simulink model "BalanceCode_MSM_Micro_20b"  (R2020b)
settings: Solver=FixedStepDiscrete  StartTime=0.0  StopTime=inf  FixedStep=TS  RelTol=1e-3  EnableMultiTasking=on
PostLoadFcn:
  | TS=.007;
undefined symbols (not defined in the file): DiscIntNeverNeededParam
libraries: arduinolib x5, svdutilitieslib x4, MinSegLibrary_MinSegMega x4, RASPlib x3, simulink x3
settings Model: FPTRunName=FPA_Reference  SimulationMode=external  SILPILModeSetting=veronly  ExtModeTrigDuration=2  Creator=Alec  LastModifiedBy=hurstj
settings DataIOCC: LimitDataPoints=on  SaveFormat=Array  ReturnWorkspaceOutputs=off
settings OptimizationCC: EnhancedBackFolding=on  PassReuseOutputArgsThreshold=0  ExpressionDepthLimit=2147483647  MaxStackSize=64  OptimizeBlockOrder=speed  DifferentSizesBufferReuse=on  OptimizationCustomize=off
settings DebuggingCC: UnderspecifiedInitializationDetection=Classic  MergeDetectMultiDrivingBlocksExec=none  ParameterPrecisionLossMsg=none  ParameterTunabilityLossMsg=error  StateNameClashWarn=warning  SFUnexpectedBacktrackingDiag=warning  SFNoUnconditionalDefaultTransitionDiag=warning  SFExecutionAtInitializationDiag=none  ArithmeticOperatorsInVariantConditions=warning
settings HardwareCC: ProdBitPerInt=16  ProdBitPerPointer=16  ProdBitPerSizeT=16  ProdBitPerPtrDiffT=16  ProdLargestAtomicFloat=None  ProdWordSize=8  ProdHWDeviceType=Atmel->AVR  UseEmbeddedCoderFeatures=off  UseSimulinkCoderFeatures=off
settings ModelReferenceCC: PropagateSignalLabelsOutOfModel=off
settings SFSimCC: SimUseLocalCustomCode=off  MATLABDynamicMemAlloc=off  CustomCodeUndefinedFunction=UseInterfaceOnly
settings RTWCC: Description=Embedded Coder  SystemTargetFile=ert.tlc  HardwareBoard=Arduino Mega 2560  TemplateMakefile=ert_default_tmf  RTWVerbose=off  RTWUseLocalCustomCode=off  Toolchain=Arduino AVR  BuildConfiguration=Faster Runs
settings CodeAppCC: ForceParamTrailComments=on  OperatorAnnotations=on
settings ERTTargetCC: ERTCustomFileBanners=off  SupportContinuousTime=on  SupportNonInlinedSFcns=on  RemoveResetFunc=off  SupportVariableSizeSignals=on  ModelStepFunctionPrototypeControlCompliant=off  ExtModeStaticAllocSize=2048
settings ConfigComp: CovMetricSettings=dw  CovSaveCumulativeToWorkspaceVar=on  CovSaveSingleToWorkspaceVar=on  CovExternalEMLEnable=off

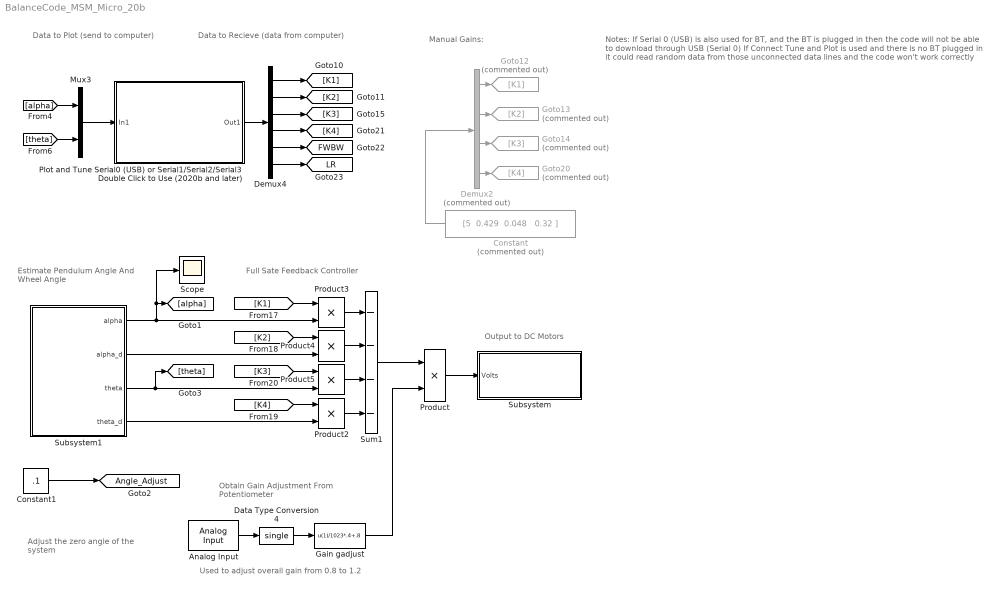
== system BalanceCode_MSM_Micro_20b ==
  note: Notes:
      |
      | If Serial 0 (USB) is also used for BT, and the BT is plugged in then the code will not be able to download through USB (Serial 0)
      |
      | If Connect Tune and Plot is used and there is no BT plugged in it could read random data from those unconnected data lines and the code won't work correctly
  note: Estimate Pendulum Angle
      | And Wheel Angle
  note: Full Sate Feedback Controller
  note: Manual Gains:
  note: Obtain Gain Adjustment
      | From Potentiometer
  note: Output to DC Motors
  note: Used to adjust overall gain from 0.8 to 1.2
  note: Adjust the zero angle
      | of the system
  note: Data to Plot
      | (send to computer)
  note: Data to Recieve
      | (data from computer)
  Analog Input : arduinolib/Analog Input  pinNumber=13  ReadResultsOnly=off  ConversionTriggerSource=Software  ExternalTriggerType=uint32( 0 )  OutputDataType=uint16  EnableConversionCompleteNotify=off  EnableOuputStatus=off  SampleTime=-1  blockPlatform=arduino
  Constant : Constant  Commented=on  Value="[5  0.429  0.048   0.32 ]"  OutDataTypeStr=single
  Constant1 : Constant  Value=.1
  Data Type Conversion4 : DataTypeConversion  OutDataTypeStr=single
  Demux2 : Demux  Commented=on
  Demux4 : Demux  Outputs=6
  Gain gadjust : Fcn  Expr=u(1)/1023*.4+.8
  Goto12 : Goto  Commented=on  GotoTag=K1
  Goto13 : Goto  Commented=on  GotoTag=K2
  Goto14 : Goto  Commented=on  GotoTag=K3
  Goto20 : Goto  Commented=on  GotoTag=K4
  Mux3 : Mux  Inputs=2
  Plot and Tune Serial0 (USB) or Serial1/Serial2/Serial3 Double Click to Use (2020b and later) : Subsystem  mask{COMport=6, Ard_Serial=3, ConnectText=<<<<<  CONNECTED  >>>>>><<<<<  CONNECTED  >>>>>><<<<<  CONNECTED  >>>>>><<<<<  CONNECTED  >>>>>>, NData=6, Data0=[7.73  0.42  0.048  0.32  0  0], DSend=[7.73  0.42  0.048  0.32  0  0], Ncx=2, NumSamples=500, Parameter10=10, Parameter12=10, Parameter13=}
      mask prompts: COMport "COM Port: (device manager)"; Ard_Serial "Arduino Serial: (0 - 3)"; NData "#  Variables:"; Data0 "Initial Values:"; DSend "Data to Send:"; Ncx "# Variables:"; NumSamples "# Samples:"; Parameter10 "OnSettingChange"; Parameter12 "OnSettingChange 2"; Parameter13 "MSM9V:  [4.8341    0.2684    0.03    0.2 0 0]*0"
      mask Callback DSend: evalin('base','if(exist(''COMdevice'')),write(COMdevice,str2num(get_param(gcb,''Dsend'')),"single"),end')
      mask Callback Parameter10: set_param(gcb,'Parameter10','10')
      mask Callback Parameter12: set_param(gcb,'Parameter12','10')
      mask DialogControl DescGroupVar Prompt: Send data to/from computer to COM device.
      mask DialogControl Control9 Prompt: Connect to COM device (Microcontroller or BT).  Can press TAB to send data in the Data to Send dialog box.  Arduino Serial 0 is USB
      mask DialogControl Control3 Prompt: Connect to COM port
      mask DialogControl Control3 Callback:
      | if(evalin('base','exist(''COMdevice'')')),
      |     disp('COM port already connected');
      | else
      |    evalin('base','COMdevice=serialport([''COM'' get_param(gcb,''COMport'')],115200)')
      | end
      | set_param(gcb,'Parameter10','1')
      mask DialogControl Control6 Prompt: Disconnect COM port
      mask DialogControl Control6 Callback:
      | evalin('base','if(exist(''COMdevice'')), disp(''Closing COM port''),clear(''COMdevice''),end')
      | set_param(gcb,'Parameter10','0')
      mask DialogControl ParameterGroupVar Prompt: Tune/Recieve - Properties of Data from Computer to Microcontroller (single data type only):
      mask DialogControl Control2 Prompt: Click to Send Data
      mask DialogControl Control2 Callback:
      | %evalin('base','write(COMdevice,30,"single")')
      | evalin('base','write(COMdevice,str2num(get_param(gcb,''Dsend'')),"single")')
      mask DialogControl Container7 Prompt: Plot/Save - Properties of Data from Microntroller to Plot/Save (single data type only)
      mask DialogControl Control7 Prompt: Click to Plot Data
      mask DialogControl Control7 Callback:
      | evalin('base','if(exist(''COMdevice'')), disp(''COM port open''),else, disp(''Opening COM Port''),end')
      | set_param(gcb,'Parameter12','10') % force mask draw
      | SerialPlot_20b_Timer(['COM' get_param(gcb,'COMport')], 'single', str2num(get_param(gcb,'NumSamples')), 115200,str2num(get_param(gcb,'Ncx')))
      | set_param(gcb,'Parameter12','11') % force mask draw
      mask DialogControl Control12 Prompt: [19 0.7 0 .19]
      mask Display:
      | text(15,75,'Serial Connect Tune')
      | text(45,60,'and Plot')
      | text(35,36,'Serial Status:')
      | 
      | if(evalin('base','exist(''COMdevice'')'))
      | 
      |     patch([0 0 300 300], [0 300 300 0],[0 1 0])
      |     text(15,75,'Serial Connect Tune')
      |     text(45,60,'and Plot')
      |     text(35,36,'Serial Status:')
      |     text(0,16,'<<<  CONNECTED  >>>>')
      |     %set_param(gcb,'ConnectText','<<<<<  CONNECTED  >>>>>><<<<<  CONNECTED  >>>>>><<<<<  CONNECTED  >>>>>><<<<<  CONNECTED  >>>>>>')
      | 
      | else
      |     text(4,16,'- - - - disconnected - - - -')
      |     %set_param(gcb,'ConnectText','- - - - - - disconnected - - - - - -- - - - - - disconnected - - - - - -- - - - - - disconnected - - - - - -- - - - - - disconnected - - - - - -- - - - - - disconnected - - - - - -')
      | end
  Product : Product  RndMeth=Zero
  Product{2..5} (4 alike) : Product
  Scope : Scope
  Subsystem : Subsystem  mask{Vsupply=7.8}
      mask prompts: Vsupply "Driver Supply Voltage"
      mask DialogControl DescGroupVar Prompt: Voltage to Motor
      mask DialogControl DescTextVar Prompt: Applies the same voltage to both motors.  No Independent control available.
      mask DialogControl ParameterGroupVar Prompt: Parameters:
      mask DialogControl Control2 Prompt: Voltage available to motor driver.  Reasonable values are 4.9 for USB, and 7.6 for a 9V battery.
      mask Display:
      | %fprintf('Volts to')
      | %fprintf(['\n\n Motors'])
      | text(35,35, 'Volts to Motor')
      | text(35,20,['Vsupply=' num2str(Vsupply)])
  Subsystem1 : Subsystem  mask{GBiasMask=0}
      mask prompts: GBiasMask "Gyro Bias (0 will calibrate automatically)"
      mask DialogControl DescGroupVar Prompt: Estimate Pendulum and Wheel Angle
      mask DialogControl DescTextVar Prompt: Estimate pendulum angle from gyroscope and acclerometer using complimentary filter.  Absolute wheel position and velocity from Encoder and Pendulum.
      mask DialogControl ParameterGroupVar Prompt: Parameters (Fixed, Non-Editable)
      mask Display:
      | fprintf('State')
      | fprintf(['\n\n Estimation'])
  Sum1 : Sum  Inputs=----
  tag scope: Angle_Adjust=global, FWBW=global, LR=global
  wires:
  Product2/1 -> Sum1/4
  Product3/1 -> Sum1/1
  Gain gadjust/1 -> Product/2
  Constant/1 -> Demux2/1
  Analog Input/1 -> Data Type Conversion4/1
  Demux2/1 -> Goto12/1
  Demux2/2 -> Goto13/1
  Product4/1 -> Sum1/2
  Data Type Conversion4/1 -> Gain gadjust/1
  Subsystem1/4(theta_d) -> Product2/2
  [K1] -> Product3/1
  Demux2/3 -> Goto14/1
  Sum1/1 -> Product/1
  Product5/1 -> Sum1/3
  [K4] -> Product2/1
  [K3] -> Product5/1
  Subsystem1/3(theta) -> [theta], Product5/2
  Demux2/4 -> Goto20/1
  [K2] -> Product4/1
  Subsystem1/2(alpha_d) -> Product4/2
  Constant1/1 -> [Angle_Adjust]
  Product/1 -> Subsystem/1(Volts)
  Subsystem1/1(alpha) -> Product3/2, Scope/1, [alpha]
  [theta] -> Mux3/2
  [alpha] -> Mux3/1
  Mux3/1 -> Plot and Tune Serial0 (USB) or Serial1/Serial2/Serial3 Double Click to Use (2020b and later)/1(In1)
  Plot and Tune Serial0 (USB) or Serial1/Serial2/Serial3 Double Click to Use (2020b and later)/1(Out1) -> Demux4/1
  Demux4/6 -> [LR]
  Demux4/1 -> [K1]
  Demux4/2 -> [K2]
  Demux4/3 -> [K3]
  Demux4/4 -> [K4]
  Demux4/5 -> [FWBW]

== system BalanceCode_MSM_Micro_20b/Plot and Tune Serial0 (USB) or Serial1//Serial2//Serial3 Double Click to Use (2020b and later) ==
  In1 : Inport
  MATLAB System : RASPlib/Double Click to Plot Serial Data/MATLAB System  is_post_2015a=~verLessThan( 'matlab', '8.6' )
      settings: SourceProductName=Rensselaer Arduino Support Package
  Send/Recieve to Serial0/Serial1/Serial2/Serial3 : Subsystem  Variant=on
  Terminator : Terminator
  Out1 : Outport
  wires:
  MATLAB System/1 -> Terminator/1
  In1/1 -> Send/Recieve to Serial0/Serial1/Serial2/Serial3/1(In1)
  Send/Recieve to Serial0/Serial1/Serial2/Serial3/1(Out1) -> Out1/1

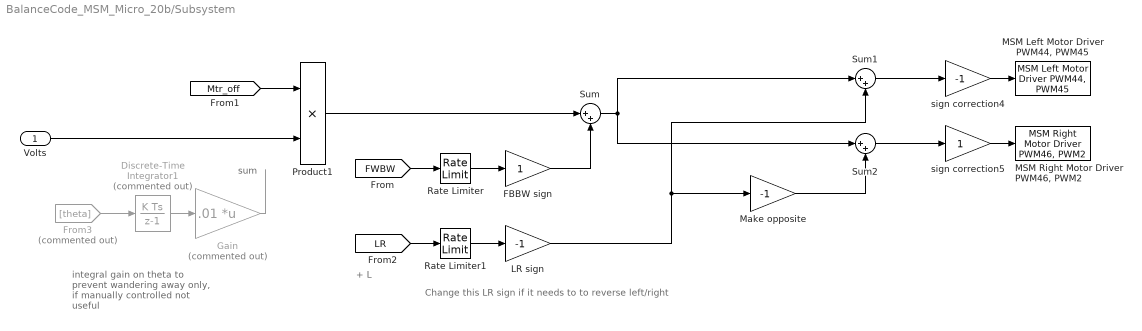
== system BalanceCode_MSM_Micro_20b/Subsystem ==
  note: sum
  note: integral gain on theta to prevent wandering away only, if manually controlled not useful
  note: Change this LR sign if it needs to to reverse left/right
  note: + L
  Volts : Inport
  Discrete-Time Integrator1 : DiscreteIntegrator  Commented=on  SampleTime=TS  ICPrevOutput=DiscIntNeverNeededParam  ICPrevScaledInput=DiscIntNeverNeededParam
  FBBW sign : Gain  OutDataTypeStr=single
  From3 : From  Commented=on  GotoTag=theta
  Gain : Gain  Commented=on  Gain=.01  Multiplication=Matrix(K*u)
  LR sign : Gain  Gain=-1  OutDataTypeStr=single
  "MSM Left Motor Driver PWM44, PWM45" : MinSegLibrary_MinSegMega/MSM Left Motor Driver PWM44, PWM45  Vsupply=Vsupply  PWMoffset=0
      settings: SourceProductName=Rensselaer Arduino Support Package
  "MSM Right Motor Driver PWM46, PWM2 " : MinSegLibrary_MinSegMega/MSM Right Motor Driver PWM46, PWM2   Vsupply=Vsupply  PWMoffset=0
      settings: SourceProductName=Rensselaer Arduino Support Package
  "Make opposite " : Gain  Gain=-1  OutDataTypeStr=single
  Product1 : Product  RndMeth=Zero
  Rate Limiter : RateLimiter  RisingSlewLimit=2  FallingSlewLimit=-2  SampleTimeMode=inherited
  Rate Limiter1 : RateLimiter  RisingSlewLimit=2  FallingSlewLimit=-2  SampleTimeMode=inherited
  Sum : Sum  Inputs=|++
  Sum1 : Sum  Inputs=|++
  Sum2 : Sum  Inputs=|++
  sign correction4 : Gain  Gain=-1  OutDataTypeStr=single
  sign correction5 : Gain  OutDataTypeStr=single
  wires:
  Volts/1 -> Product1/2
  From3/1 -> Discrete-Time Integrator1/1
  Gain/1 -> ?
  [Mtr_off] -> Product1/1
  Discrete-Time Integrator1/1 -> Gain/1
  Product1/1 -> Sum/1
  [FWBW] -> Rate Limiter/1
  Rate Limiter/1 -> FBBW sign/1
  [LR] -> Rate Limiter1/1
  Rate Limiter1/1 -> LR sign/1
  Sum/1 -> Sum2/1, Sum1/1
  sign correction5/1 -> "MSM Right Motor Driver PWM46, PWM2 "/1
  sign correction4/1 -> "MSM Left Motor Driver PWM44, PWM45"/1
  Sum1/1 -> sign correction4/1
  Sum2/1 -> sign correction5/1
  "Make opposite "/1 -> Sum2/2
  LR sign/1 -> "Make opposite "/1, Sum1/2
  FBBW sign/1 -> Sum/2

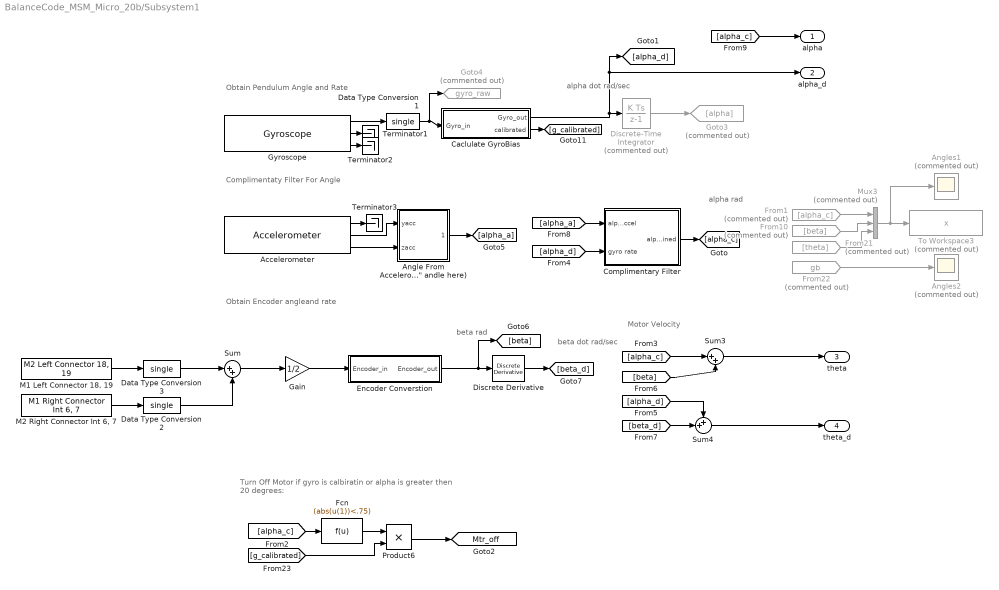
== system BalanceCode_MSM_Micro_20b/Subsystem1 ==
  note: Complimentaty Filter For Angle
  note: alpha dot
      | rad/sec
  note: alpha
      | rad
  note: Motor Velocity
  note: Turn Off Motor if gyro is calbiratin or
      | alpha is greater then 20 degrees:
  note: Obtain Pendulum Angle and Rate
  note: beta dot
      | rad/sec
  note: beta
      | rad
  note: Obtain Encoder angleand rate
  " Complimentary Filter" : Subsystem
  Accelerometer : RASPlib/Accelerometer  SimulateUsing=Code generation
      settings: SourceProductName=Rensselaer Arduino Support Package
  "Angle From Accelerometer (adjust \"zero\" andle here)" : Subsystem
  Angles1 : Scope  Commented=on
  Angles2 : Scope  Commented=on
  Caclulate GyroBias : Subsystem  mask{GSm=.00013316}
      mask DialogControl DescGroupVar Prompt: Calibrate Gyroscope
      mask DialogControl DescTextVar Prompt: Estimates gyro bias from during fist 1 second of operation.  It is important that the system is NOT moving during the fist 1 second.
      mask DialogControl ParameterGroupVar Prompt: Paramters (non tunable):
      mask DialogControl Control2 Prompt: Gyro Bias (Calibrated Automatically)
      mask DialogControl Control3 Prompt: Unit Conversion (Fixed)
  Data Type Conversion1 : DataTypeConversion  OutDataTypeStr=single
  Data Type Conversion2 : DataTypeConversion  OutDataTypeStr=single
  Data Type Conversion3 : DataTypeConversion  OutDataTypeStr=single
  Discrete Derivative : simulink/Discrete/Discrete Derivative  gainval=1.0  ICPrevScaledInput=0.0  OutMin=[]  OutMax=[]  OutDataType=fixdt(1, 16)  OutScaling=2^-10  DoSatur=off
  Discrete-Time Integrator : DiscreteIntegrator  Commented=on  SampleTime=TS  ICPrevOutput=DiscIntNeverNeededParam  ICPrevScaledInput=DiscIntNeverNeededParam
  Encoder Converstion : Subsystem  mask{ESm=0.0047}
      mask DialogControl DescGroupVar Prompt: Encoder Unit Converstion
      mask DialogControl ParameterGroupVar Prompt: Paramters (non tunable):
      mask DialogControl Control2 Prompt: Unit Conversion (Fixed)
  Fcn : Fcn  Expr=(abs(u(1))<.75)
  From1 : From  Commented=on  GotoTag=alpha_c
  From10 : From  Commented=on  GotoTag=beta
  From21 : From  Commented=on  GotoTag=theta  TagVisibility=global
  From22 : From  Commented=on  GotoTag=gb  TagVisibility=global
  Gain : Gain  Gain=1/2
  Goto3 : Goto  Commented=on  GotoTag=alpha
  Goto4 : Goto  Commented=on  GotoTag=gyro_raw  TagVisibility=global
  Gyroscope : RASPlib/Gyroscope  DLPFmode=0
      settings: SourceProductName=Rensselaer Arduino Support Package
  "M1 Left Connector 18, 19" : MinSegLibrary_MinSegMega/M2 Left Connector 18, 19  Encoder=1  PinA=18  PinB=19
      settings: SourceProductName=Rensselaer Arduino Support Package
  "M2 Right Connector Int 6, 7" : MinSegLibrary_MinSegMega/M1 Right Connector Int 6, 7  Encoder=2  PinA=6  PinB=7
      settings: SourceProductName=Rensselaer Arduino Support Package
  Mux3 : Mux  Commented=on  Inputs=3
  Product6 : Product
  Sum : Sum  Inputs=|++
  Sum3 : Sum  Inputs=|++
  Sum4 : Sum  Inputs=++|
  Terminator1 : Terminator
  Terminator2 : Terminator
  Terminator3 : Terminator
  To Workspace3 : ToWorkspace  Commented=on  VariableName=x  SampleTime=-1
      settings: Save2DSignal=2-D array (concatenate along first dimension)
  alpha : Outport
  alpha_d : Outport  Port=2
  theta : Outport  Port=3
  theta_d : Outport  Port=4
  tag scope: Mtr_off=global
  wires:
  Gyroscope/1 -> Data Type Conversion1/1
  [beta] -> Sum3/2
  Gyroscope/3 -> Terminator2/1
  [alpha_d] -> Sum4/1
  From1/1 -> Mux3/1
  Gyroscope/2 -> Terminator1/1
  [beta_d] -> Sum4/2
  [alpha_c] -> Sum3/1
  "Angle From Accelerometer (adjust \"zero\" andle here)"/1(angle rad) -> [alpha_a]
  Data Type Conversion1/1 -> Goto4/1, Caclulate GyroBias/1(Gyro_in)
  Accelerometer/3 -> "Angle From Accelerometer (adjust \"zero\" andle here)"/2(zacc)
  Discrete-Time Integrator/1 -> Goto3/1
  [alpha_a] -> " Complimentary Filter"/1(alpha accel)
  From10/1 -> Mux3/2
  From21/1 -> Mux3/3
  Accelerometer/2 -> "Angle From Accelerometer (adjust \"zero\" andle here)"/1(yacc)
  Accelerometer/1 -> Terminator3/1
  Mux3/1 -> Angles1/1, To Workspace3/1
  Caclulate GyroBias/1(Gyro_out) -> [alpha_d], alpha_d/1, Discrete-Time Integrator/1
  [alpha_d] -> " Complimentary Filter"/2(gyro rate)
  From22/1 -> Angles2/1
  Sum4/1 -> theta_d/1
  Sum3/1 -> theta/1
  Fcn/1 -> Product6/1
  Product6/1 -> [Mtr_off]
  [alpha_c] -> Fcn/1
  [g_calibrated] -> Product6/2
  Discrete Derivative/1 -> [beta_d]
  "M1 Left Connector 18, 19"/1 -> Data Type Conversion3/1
  " Complimentary Filter"/1(alpha combined) -> [alpha_c]
  [alpha_c] -> alpha/1
  Encoder Converstion/1(Encoder_out) -> [beta], Discrete Derivative/1
  Caclulate GyroBias/2(calibrated) -> [g_calibrated]
  "M2 Right Connector Int 6, 7"/1 -> Data Type Conversion2/1
  Data Type Conversion3/1 -> Sum/1
  Data Type Conversion2/1 -> Sum/2
  Sum/1 -> Gain/1
  Gain/1 -> Encoder Converstion/1(Encoder_in)

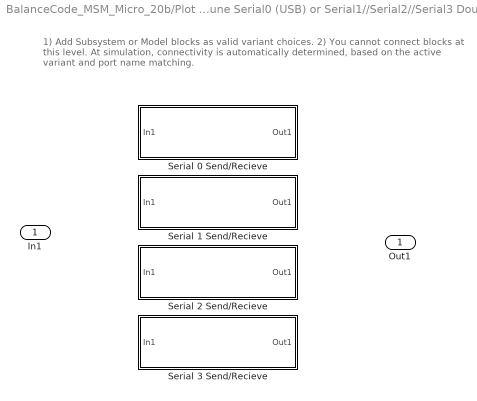
== system BalanceCode_MSM_Micro_20b/Plot and Tune Serial0 (USB) or Serial1//Serial2//Serial3 Double Click to Use (2020b and later)/Send//Recieve to Serial0//Serial1//Serial2//Serial3 ==
  note: 1) Add Subsystem or Model blocks as valid variant choices.
      | 2) You cannot connect blocks at this level. At simulation, connectivity is automatically
      | determined, based on the active variant and port name matching.
  In1 : Inport
  Serial 0 Send/Recieve : Subsystem  VariantControl=Ard_Serial==0
  Serial 1 Send/Recieve : Subsystem  VariantControl=Ard_Serial==1
  Serial 2 Send/Recieve : Subsystem  VariantControl=Ard_Serial==2
  Serial 3 Send/Recieve : Subsystem  VariantControl=Ard_Serial==3
  Out1 : Outport

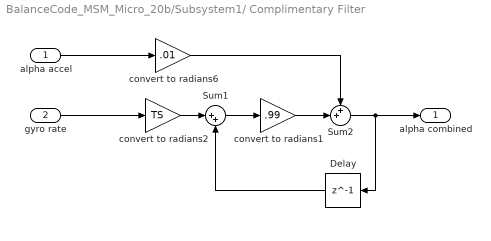
== system BalanceCode_MSM_Micro_20b/Subsystem1/ Complimentary Filter ==
  alpha accel : Inport
  gyro rate : Inport  Port=2
  Delay : Delay  DelayLength=1  SampleTime=TS
  Sum1 : Sum  Inputs=|++
  Sum2 : Sum  Inputs=++|
  convert to radians1 : Gain  Gain=.99  OutDataTypeStr=single
  convert to radians2 : Gain  Gain=TS  OutDataTypeStr=single
  convert to radians6 : Gain  Gain=.01  OutDataTypeStr=single
  alpha combined : Outport
  wires:
  gyro rate/1 -> convert to radians2/1
  Sum1/1 -> convert to radians1/1
  convert to radians6/1 -> Sum2/1
  alpha accel/1 -> convert to radians6/1
  convert to radians1/1 -> Sum2/2
  Delay/1 -> Sum1/2
  convert to radians2/1 -> Sum1/1
  Sum2/1 -> Delay/1, alpha combined/1

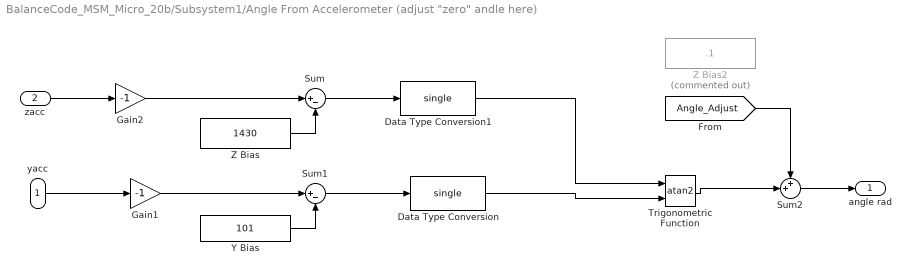
== system BalanceCode_MSM_Micro_20b/Subsystem1/Angle From Accelerometer (adjust "zero" andle here) ==
  yacc : Inport
  zacc : Inport  Port=2
  Data Type Conversion : DataTypeConversion  OutDataTypeStr=single
  Data Type Conversion1 : DataTypeConversion  OutDataTypeStr=single
  Gain1 : Gain  Gain=-1
  Gain2 : Gain  Gain=-1
  Sum : Sum  Inputs=|+-
  Sum1 : Sum  Inputs=|+-
  Sum2 : Sum  Inputs=++|
  Trigonometric Function : Trigonometry  Operator=atan2
  Y Bias : Constant  Value=101
  Z Bias : Constant  Value=1430
  Z Bias2 : Constant  Commented=on  Value=.1  OutDataTypeStr=single
  angle rad : Outport
  wires:
  Sum1/1 -> Data Type Conversion/1
  Gain2/1 -> Sum/1
  Sum/1 -> Data Type Conversion1/1
  Z Bias/1 -> Sum/2
  Gain1/1 -> Sum1/1
  Y Bias/1 -> Sum1/2
  zacc/1 -> Gain2/1
  yacc/1 -> Gain1/1
  Trigonometric Function/1 -> Sum2/2
  Sum2/1 -> angle rad/1
  [Angle_Adjust] -> Sum2/1
  Data Type Conversion1/1 -> Trigonometric Function/1
  Data Type Conversion/1 -> Trigonometric Function/2

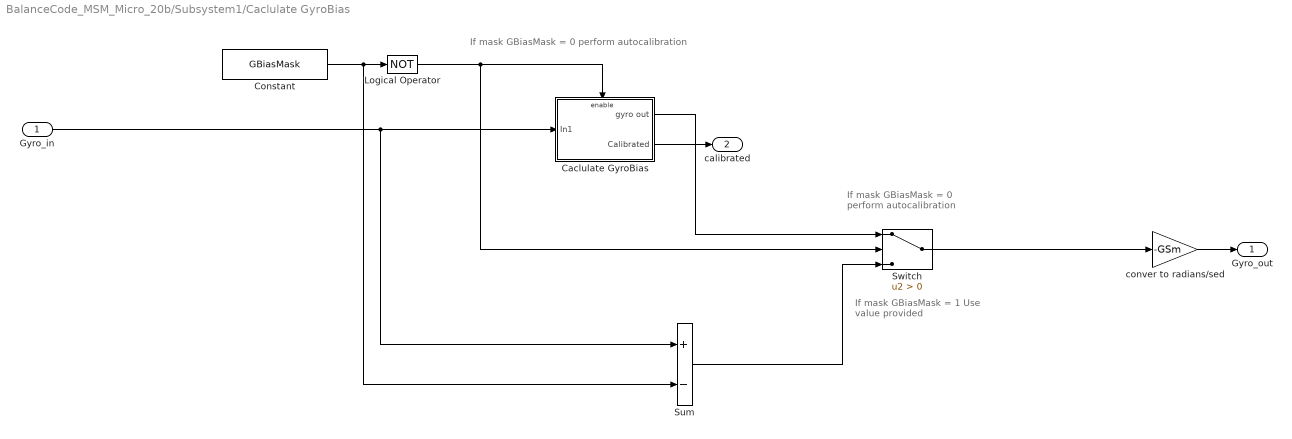
== system BalanceCode_MSM_Micro_20b/Subsystem1/Caclulate GyroBias ==
  note: If mask GBiasMask = 1
      | Use value provided
  note: If mask GBiasMask = 0 perform autocalibration
  note: If mask GBiasMask = 0
      |  perform autocalibration
  Gyro_in : Inport
  Caclulate GyroBias : Subsystem
  Constant : Constant  Value=GBiasMask
  Logical Operator : Logic  Operator=NOT  AllPortsSameDT=off  OutDataTypeStr=boolean
  Sum : Sum  Inputs=+-
  Switch : Switch  Criteria=u2 > Threshold
  conver to radians/sed : Gain  Gain=-GSm  OutDataTypeStr=single
  Gyro_out : Outport
  calibrated : Outport  Port=2
  wires:
  conver to radians/sed/1 -> Gyro_out/1
  Switch/1 -> conver to radians/sed/1
  Logical Operator/1 -> Switch/2, Caclulate GyroBias/Enable
  Constant/1 -> Sum/2, Logical Operator/1
  Sum/1 -> Switch/3
  Gyro_in/1 -> Caclulate GyroBias/1(In1), Sum/1
  Caclulate GyroBias/1(gyro out) -> Switch/1
  Caclulate GyroBias/2(Calibrated) -> calibrated/1

== system BalanceCode_MSM_Micro_20b/Subsystem1/Encoder Converstion ==
  Encoder_in : Inport
  convert to radians : Gain  Gain=-ESm  OutDataTypeStr=single
  Encoder_out : Outport
  wires:
  Encoder_in/1 -> convert to radians/1
  convert to radians/1 -> Encoder_out/1

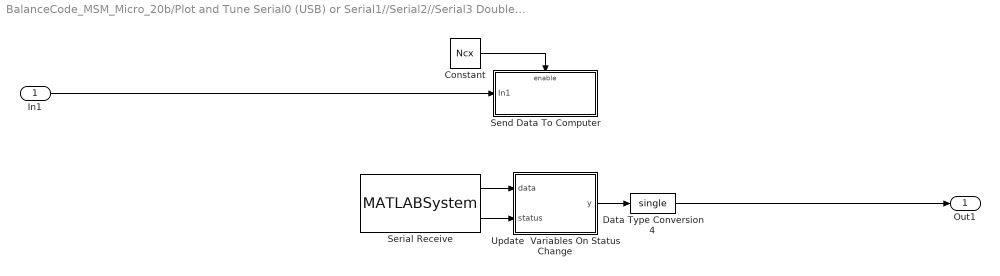
== system BalanceCode_MSM_Micro_20b/Plot and Tune Serial0 (USB) or Serial1//Serial2//Serial3 Double Click to Use (2020b and later)/Send//Recieve to Serial0//Serial1//Serial2//Serial3/Serial 0 Send//Recieve ==
  In1 : Inport
  Constant : Constant  Value=Ncx
  Data Type Conversion4 : DataTypeConversion  OutDataTypeStr=single
  Send Data To Computer : Subsystem  TreatAsAtomicUnit=on
  Serial Receive : MATLABSystem  InitFcn=|  System=codertarget.arduinobase.internal.arduino_SerialRead  isARMArch=off  portNumber=portNumber  SampleTime=SampleTime  DataType=double  Datalength=Datalength  Protocol=0  mask(Arduino Serial Receive){isARMArch=off, portNumber=0, DataType=double, Datalength=NData, SampleTime=TS, showOutStatus=on, blockPlatform=arduino}
      | %codertarget.arduinobase.blocks.arduinoBlockInitFcnCallback(gcbh);
      | %codertarget.arduinobase.blocks.registerSerialBlock(gcbh);
      mask prompts: isARMArch "Is ARM Architecture"; portNumber "Port number:"; DataType "Data type:"; Datalength "Data length:"; SampleTime "Sample time:"; showOutStatus "Output receiving status"; blockPlatform "Block platform:"
      mask help:
      | Receive an [Nx1] array of data on the specified serial port and write it to the Data block output.When data is not available, write 0 to the Data block output.
      |
      | The Status port outputs 0 when the length of data received is less than the Data length specified. Otherwise, it emits 1.
      |
      | Use the Data length parameter to specify the number of data bytes  to receive.
      mask init:
      | codertarget.arduinobase.blocks.arduinoSerialReadCallback('MaskInitialization');
      mask Help: eval('codertarget.internal.helpView(''arduinoert'', ''arduinolibarduinoserialreceive'')')
      mask TypeOptions isARMArch: isARMArch
      mask Callback isARMArch: codertarget.arduinobase.blocks.arduinoSerialReadCallback('isARMArch');
      mask TypeOptions portNumber: portNumber
      mask TypeOptions DataType: DataType
      mask TypeOptions Datalength: Datalength
      mask TypeOptions SampleTime: SampleTime
      mask DialogControl Control2 Prompt: View pin map
      mask DialogControl Control2 Callback:
      | file = [codertarget.arduinobase.internal.getBaseSpPkgRootDir filesep 'blocks' filesep 'mex' filesep 'arduinoPinMapping.html'];
      | web(file)
      mask Display:
      | pic=imread('serial.png');image(pic,[0.28 0.18 0.45 0.65]);text(0.5, 0.15, 'Port 0', 'horizontalAlignment', 'center');
      | color('blue');
      | text(0.55, 0.87, 'ARDUINO', 'horizontalAlignment', 'left');
      | color('black');
      | port_label('output', 1, 'Data');
      | port_label('output', 2, 'Status');
  Update  Variables On Status Change : Subsystem
  Out1 : Outport
  wires:
  Update  Variables On Status Change/1(y) -> Data Type Conversion4/1
  In1/1 -> Send Data To Computer/1(In1)
  Constant/1 -> Send Data To Computer/Enable
  Serial Receive/2 -> Update  Variables On Status Change/2(status)
  Serial Receive/1 -> Update  Variables On Status Change/1(data)
  Data Type Conversion4/1 -> Out1/1

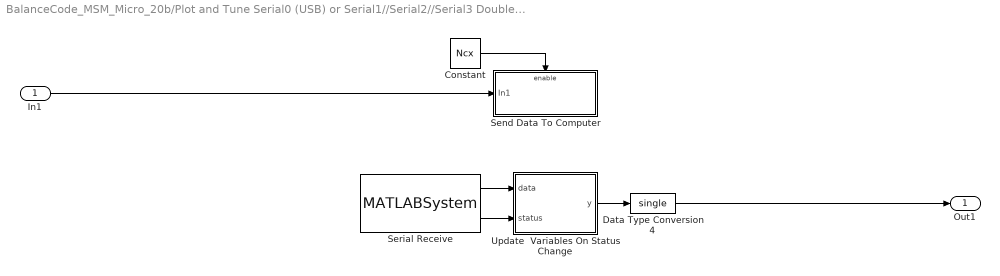
== system BalanceCode_MSM_Micro_20b/Plot and Tune Serial0 (USB) or Serial1//Serial2//Serial3 Double Click to Use (2020b and later)/Send//Recieve to Serial0//Serial1//Serial2//Serial3/Serial 1 Send//Recieve ==
  In1 : Inport
  Constant : Constant  Value=Ncx
  Data Type Conversion4 : DataTypeConversion  OutDataTypeStr=single
  Send Data To Computer : Subsystem  TreatAsAtomicUnit=on
  Serial Receive : MATLABSystem  InitFcn=|  System=codertarget.arduinobase.internal.arduino_SerialRead  isARMArch=off  portNumber=portNumber  SampleTime=SampleTime  DataType=double  Datalength=Datalength  Protocol=0  mask(Arduino Serial Receive){isARMArch=off, portNumber=1, DataType=double, Datalength=NData, SampleTime=TS, showOutStatus=on, blockPlatform=arduino}
      | %codertarget.arduinobase.blocks.arduinoBlockInitFcnCallback(gcbh);
      | %codertarget.arduinobase.blocks.registerSerialBlock(gcbh);
      mask prompts: isARMArch "Is ARM Architecture"; portNumber "Port number:"; DataType "Data type:"; Datalength "Data length:"; SampleTime "Sample time:"; showOutStatus "Output receiving status"; blockPlatform "Block platform:"
      mask help:
      | Receive an [Nx1] array of data on the specified serial port and write it to the Data block output.When data is not available, write 0 to the Data block output.
      |
      | The Status port outputs 0 when the length of data received is less than the Data length specified. Otherwise, it emits 1.
      |
      | Use the Data length parameter to specify the number of data bytes  to receive.
      mask init:
      | codertarget.arduinobase.blocks.arduinoSerialReadCallback('MaskInitialization');
      mask Help: eval('codertarget.internal.helpView(''arduinoert'', ''arduinolibarduinoserialreceive'')')
      mask TypeOptions isARMArch: isARMArch
      mask Callback isARMArch: codertarget.arduinobase.blocks.arduinoSerialReadCallback('isARMArch');
      mask TypeOptions portNumber: portNumber
      mask TypeOptions DataType: DataType
      mask TypeOptions Datalength: Datalength
      mask TypeOptions SampleTime: SampleTime
      mask DialogControl Control2 Prompt: View pin map
      mask DialogControl Control2 Callback:
      | file = [codertarget.arduinobase.internal.getBaseSpPkgRootDir filesep 'blocks' filesep 'mex' filesep 'arduinoPinMapping.html'];
      | web(file)
      mask Display:
      | pic=imread('serial.png');image(pic,[0.28 0.18 0.45 0.65]);text(0.5, 0.15, 'Port 1', 'horizontalAlignment', 'center');
      | color('blue');
      | text(0.55, 0.87, 'ARDUINO', 'horizontalAlignment', 'left');
      | color('black');
      | port_label('output', 1, 'Data');
      | port_label('output', 2, 'Status');
  Update  Variables On Status Change : Subsystem
  Out1 : Outport
  wires:
  Data Type Conversion4/1 -> Out1/1
  Serial Receive/1 -> Update  Variables On Status Change/1(data)
  Serial Receive/2 -> Update  Variables On Status Change/2(status)
  Constant/1 -> Send Data To Computer/Enable
  In1/1 -> Send Data To Computer/1(In1)
  Update  Variables On Status Change/1(y) -> Data Type Conversion4/1

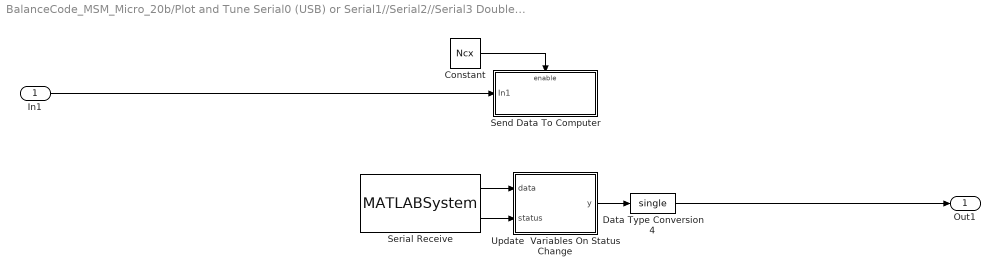
== system BalanceCode_MSM_Micro_20b/Plot and Tune Serial0 (USB) or Serial1//Serial2//Serial3 Double Click to Use (2020b and later)/Send//Recieve to Serial0//Serial1//Serial2//Serial3/Serial 2 Send//Recieve ==
  In1 : Inport
  Constant : Constant  Value=Ncx
  Data Type Conversion4 : DataTypeConversion  OutDataTypeStr=single
  Send Data To Computer : Subsystem  TreatAsAtomicUnit=on
  Serial Receive : MATLABSystem  InitFcn=|  System=codertarget.arduinobase.internal.arduino_SerialRead  isARMArch=off  portNumber=portNumber  SampleTime=SampleTime  DataType=double  Datalength=Datalength  Protocol=0  mask(Arduino Serial Receive){isARMArch=off, portNumber=2, DataType=double, Datalength=NData, SampleTime=TS, showOutStatus=on, blockPlatform=arduino}
      | %codertarget.arduinobase.blocks.arduinoBlockInitFcnCallback(gcbh);
      | %codertarget.arduinobase.blocks.registerSerialBlock(gcbh);
      mask prompts: isARMArch "Is ARM Architecture"; portNumber "Port number:"; DataType "Data type:"; Datalength "Data length:"; SampleTime "Sample time:"; showOutStatus "Output receiving status"; blockPlatform "Block platform:"
      mask help:
      | Receive an [Nx1] array of data on the specified serial port and write it to the Data block output.When data is not available, write 0 to the Data block output.
      |
      | The Status port outputs 0 when the length of data received is less than the Data length specified. Otherwise, it emits 1.
      |
      | Use the Data length parameter to specify the number of data bytes  to receive.
      mask init:
      | codertarget.arduinobase.blocks.arduinoSerialReadCallback('MaskInitialization');
      mask Help: eval('codertarget.internal.helpView(''arduinoert'', ''arduinolibarduinoserialreceive'')')
      mask TypeOptions isARMArch: isARMArch
      mask Callback isARMArch: codertarget.arduinobase.blocks.arduinoSerialReadCallback('isARMArch');
      mask TypeOptions portNumber: portNumber
      mask TypeOptions DataType: DataType
      mask TypeOptions Datalength: Datalength
      mask TypeOptions SampleTime: SampleTime
      mask DialogControl Control2 Prompt: View pin map
      mask DialogControl Control2 Callback:
      | file = [codertarget.arduinobase.internal.getBaseSpPkgRootDir filesep 'blocks' filesep 'mex' filesep 'arduinoPinMapping.html'];
      | web(file)
      mask Display:
      | pic=imread('serial.png');image(pic,[0.28 0.18 0.45 0.65]);text(0.5, 0.15, 'Port 2', 'horizontalAlignment', 'center');
      | color('blue');
      | text(0.55, 0.87, 'ARDUINO', 'horizontalAlignment', 'left');
      | color('black');
      | port_label('output', 1, 'Data');
      | port_label('output', 2, 'Status');
  Update  Variables On Status Change : Subsystem
  Out1 : Outport
  wires:
  Update  Variables On Status Change/1(y) -> Data Type Conversion4/1
  In1/1 -> Send Data To Computer/1(In1)
  Constant/1 -> Send Data To Computer/Enable
  Serial Receive/2 -> Update  Variables On Status Change/2(status)
  Serial Receive/1 -> Update  Variables On Status Change/1(data)
  Data Type Conversion4/1 -> Out1/1

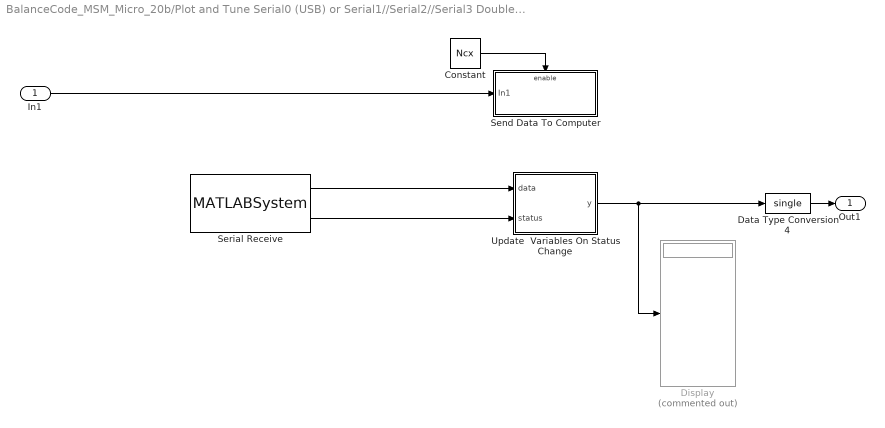
== system BalanceCode_MSM_Micro_20b/Plot and Tune Serial0 (USB) or Serial1//Serial2//Serial3 Double Click to Use (2020b and later)/Send//Recieve to Serial0//Serial1//Serial2//Serial3/Serial 3 Send//Recieve ==
  In1 : Inport
  Constant : Constant  Value=Ncx
  Data Type Conversion4 : DataTypeConversion  OutDataTypeStr=single
  Display : Display  Commented=on
  Send Data To Computer : Subsystem  TreatAsAtomicUnit=on
  Serial Receive : MATLABSystem  InitFcn=|  System=codertarget.arduinobase.internal.arduino_SerialRead  isARMArch=off  portNumber=portNumber  SampleTime=SampleTime  DataType=double  Datalength=Datalength  Protocol=0  mask(Arduino Serial Receive){isARMArch=off, portNumber=3, DataType=double, Datalength=NData, SampleTime=TS, showOutStatus=on, blockPlatform=arduino}
      | %codertarget.arduinobase.blocks.arduinoBlockInitFcnCallback(gcbh);
      | %codertarget.arduinobase.blocks.registerSerialBlock(gcbh);
      mask prompts: isARMArch "Is ARM Architecture"; portNumber "Port number:"; DataType "Data type:"; Datalength "Data length:"; SampleTime "Sample time:"; showOutStatus "Output receiving status"; blockPlatform "Block platform:"
      mask help:
      | Receive an [Nx1] array of data on the specified serial port and write it to the Data block output.When data is not available, write 0 to the Data block output.
      |
      | The Status port outputs 0 when the length of data received is less than the Data length specified. Otherwise, it emits 1.
      |
      | Use the Data length parameter to specify the number of data bytes  to receive.
      mask init:
      | codertarget.arduinobase.blocks.arduinoSerialReadCallback('MaskInitialization');
      mask Help: eval('codertarget.internal.helpView(''arduinoert'', ''arduinolibarduinoserialreceive'')')
      mask TypeOptions isARMArch: isARMArch
      mask Callback isARMArch: codertarget.arduinobase.blocks.arduinoSerialReadCallback('isARMArch');
      mask TypeOptions portNumber: portNumber
      mask TypeOptions DataType: DataType
      mask TypeOptions Datalength: Datalength
      mask TypeOptions SampleTime: SampleTime
      mask DialogControl Control2 Prompt: View pin map
      mask DialogControl Control2 Callback:
      | file = [codertarget.arduinobase.internal.getBaseSpPkgRootDir filesep 'blocks' filesep 'mex' filesep 'arduinoPinMapping.html'];
      | web(file)
      mask Display:
      | pic=imread('serial.png');image(pic,[0.28 0.18 0.45 0.65]);text(0.5, 0.15, 'Port 3', 'horizontalAlignment', 'center');
      | color('blue');
      | text(0.55, 0.87, 'ARDUINO', 'horizontalAlignment', 'left');
      | color('black');
      | port_label('output', 1, 'Data');
      | port_label('output', 2, 'Status');
  Update  Variables On Status Change : Subsystem
  Out1 : Outport
  wires:
  Update  Variables On Status Change/1(y) -> Data Type Conversion4/1, Display/1
  Serial Receive/1 -> Update  Variables On Status Change/1(data)
  Data Type Conversion4/1 -> Out1/1
  Serial Receive/2 -> Update  Variables On Status Change/2(status)
  Constant/1 -> Send Data To Computer/Enable
  In1/1 -> Send Data To Computer/1(In1)

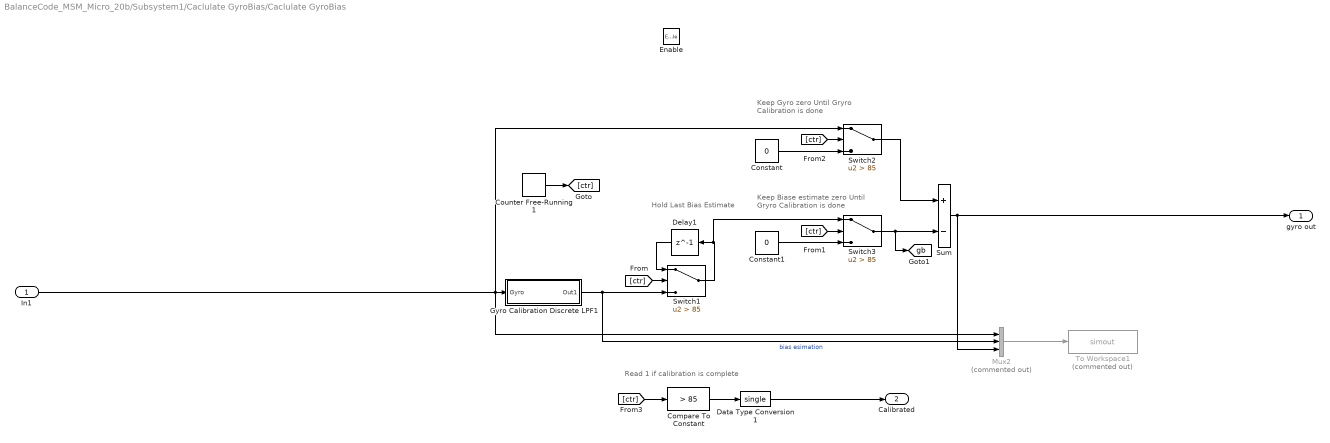
== system BalanceCode_MSM_Micro_20b/Subsystem1/Caclulate GyroBias/Caclulate GyroBias ==
  note: Keep Biase estimate zero
      | Until Gryro Calibration is done
  note: Hold Last
      | Bias Estimate
  note: Keep Gyro zero
      | Until Gryro Calibration is done
  note: Read 1 if calibration is complete
  In1 : Inport
  Enable : EnablePort
  Compare To Constant : simulink/Logic and Bit Operations/Compare To Constant  relop=>  const=85  OutDataTypeStr=boolean
  Constant : Constant  Value=0  OutDataTypeStr=single
  Constant1 : Constant  Value=0  OutDataTypeStr=single
  Counter Free-Running1 : simulink/Sources/Counter Free-Running  NumBits=32  tsamp=TS
  Data Type Conversion1 : DataTypeConversion  OutDataTypeStr=single
  Delay1 : Delay  DelayLength=1
  Gyro Calibration Discrete LPF1 : Subsystem
  Mux2 : Mux  Commented=on  Inputs=3
  Sum : Sum  Inputs=+-
  Switch1 : Switch  Criteria=u2 > Threshold  Threshold=85
  Switch2 : Switch  Criteria=u2 > Threshold  Threshold=85
  Switch3 : Switch  Criteria=u2 > Threshold  Threshold=85
  To Workspace1 : ToWorkspace  Commented=on  VariableName=simout  SampleTime=-1
      settings: Save2DSignal=2-D array (concatenate along first dimension)
  gyro out : Outport
  Calibrated : Outport  Port=2
  tag scope: gb=global
  wires:
  Switch3/1 -> [gb], Sum/2
  In1/1 -> Mux2/1, Switch2/1, Gyro Calibration Discrete LPF1/1(Gyro)
  Constant/1 -> Switch2/3
  [ctr] -> Switch3/2
  Counter Free-Running1/1 -> [ctr]
  Compare To Constant/1 -> Data Type Conversion1/1
  Sum/1 -> gyro out/1, Mux2/3
  Switch1/1 -> Switch3/1, Delay1/1
  Gyro Calibration Discrete LPF1/1(Out1) -> Mux2/2, Switch1/3  "bias esimation"
  Switch2/1 -> Sum/1
  Constant1/1 -> Switch3/3
  Data Type Conversion1/1 -> Calibrated/1
  Delay1/1 -> Switch1/1
  [ctr] -> Switch2/2
  Mux2/1 -> To Workspace1/1
  [ctr] -> Compare To Constant/1
  [ctr] -> Switch1/2

== system BalanceCode_MSM_Micro_20b/Plot and Tune Serial0 (USB) or Serial1//Serial2//Serial3 Double Click to Use (2020b and later)/Send//Recieve to Serial0//Serial1//Serial2//Serial3/Serial 0 Send//Recieve/Send Data To Computer ==
  In1 : Inport
  Enable : EnablePort
  Byte Pack : svdutilitieslib/Byte Pack  maskPackedDataType=uint8  datatypes={'single'}  byteAlign=1  blockPlatform=arduinoert
      settings: SourceProductBaseCode=ANDROID,ARDUINO,ML_ARDUINO,ECCORTEXA,ECCORTEXR,SC_BEAGLEBONE_BLUE,EC_FREEDOM_BOARD,EC_FRDM_K64F,INTEL_BLOCKSET,JETSONCPU,MICROBIT,NUCLEO,NVIDIA,PX4AUTOPILOTS,RASPPIIO,STMICRODIS,TIC2000,XILINX_BLOCKSET
  Data Type Conversion1 : DataTypeConversion  OutDataTypeStr=single
  Serial Transmit : arduinolib/Serial Transmit  portNumber=0  sendmode=write  sendformat=Decimal  floatprecision=2  blockPlatform=arduino
  wires:
  Byte Pack/1 -> Serial Transmit/1
  Data Type Conversion1/1 -> Byte Pack/1
  In1/1 -> Data Type Conversion1/1

== system BalanceCode_MSM_Micro_20b/Plot and Tune Serial0 (USB) or Serial1//Serial2//Serial3 Double Click to Use (2020b and later)/Send//Recieve to Serial0//Serial1//Serial2//Serial3/Serial 0 Send//Recieve/Update  Variables On Status Change ==
  data : Inport
  status : Inport  Port=2
  Delay : Delay  DelayLength=1  InitialCondition=Data0
  MATLAB Function1 : MATLAB Function  TreatAsAtomicUnit=on
  y : Outport
  wires:
  Delay/1 -> MATLAB Function1/2(prev_data)
  MATLAB Function1/1(y) -> Delay/1, y/1
  data/1 -> MATLAB Function1/1(data)
  status/1 -> MATLAB Function1/3(status)

== system BalanceCode_MSM_Micro_20b/Plot and Tune Serial0 (USB) or Serial1//Serial2//Serial3 Double Click to Use (2020b and later)/Send//Recieve to Serial0//Serial1//Serial2//Serial3/Serial 1 Send//Recieve/Send Data To Computer ==
  In1 : Inport
  Enable : EnablePort
  Byte Pack : svdutilitieslib/Byte Pack  maskPackedDataType=uint8  datatypes={'single'}  byteAlign=1  blockPlatform=arduinoert
      settings: SourceProductBaseCode=ANDROID,ARDUINO,ML_ARDUINO,ECCORTEXA,ECCORTEXR,SC_BEAGLEBONE_BLUE,EC_FREEDOM_BOARD,EC_FRDM_K64F,INTEL_BLOCKSET,JETSONCPU,MICROBIT,NUCLEO,NVIDIA,PX4AUTOPILOTS,RASPPIIO,STMICRODIS,TIC2000,XILINX_BLOCKSET
  Data Type Conversion1 : DataTypeConversion  OutDataTypeStr=single
  Serial Transmit : arduinolib/Serial Transmit  portNumber=1  sendmode=write  sendformat=Decimal  floatprecision=2  blockPlatform=arduino
  wires:
  In1/1 -> Data Type Conversion1/1
  Data Type Conversion1/1 -> Byte Pack/1
  Byte Pack/1 -> Serial Transmit/1

== system BalanceCode_MSM_Micro_20b/Plot and Tune Serial0 (USB) or Serial1//Serial2//Serial3 Double Click to Use (2020b and later)/Send//Recieve to Serial0//Serial1//Serial2//Serial3/Serial 1 Send//Recieve/Update  Variables On Status Change ==
  data : Inport
  status : Inport  Port=2
  Delay : Delay  DelayLength=1  InitialCondition=Data0  SampleTime=TS
  MATLAB Function1 : MATLAB Function  TreatAsAtomicUnit=on
  y : Outport
  wires:
  status/1 -> MATLAB Function1/3(status)
  data/1 -> MATLAB Function1/1(data)
  MATLAB Function1/1(y) -> y/1, Delay/1
  Delay/1 -> MATLAB Function1/2(prev_data)

== system BalanceCode_MSM_Micro_20b/Plot and Tune Serial0 (USB) or Serial1//Serial2//Serial3 Double Click to Use (2020b and later)/Send//Recieve to Serial0//Serial1//Serial2//Serial3/Serial 2 Send//Recieve/Send Data To Computer ==
  In1 : Inport
  Enable : EnablePort
  Byte Pack : svdutilitieslib/Byte Pack  maskPackedDataType=uint8  datatypes={'single'}  byteAlign=1  blockPlatform=arduinoert
      settings: SourceProductBaseCode=ANDROID,ARDUINO,ML_ARDUINO,ECCORTEXA,ECCORTEXR,SC_BEAGLEBONE_BLUE,EC_FREEDOM_BOARD,EC_FRDM_K64F,INTEL_BLOCKSET,JETSONCPU,MICROBIT,NUCLEO,NVIDIA,PX4AUTOPILOTS,RASPPIIO,STMICRODIS,TIC2000,XILINX_BLOCKSET
  Data Type Conversion1 : DataTypeConversion  OutDataTypeStr=single
  Serial Transmit : arduinolib/Serial Transmit  portNumber=2  sendmode=write  sendformat=Decimal  floatprecision=2  blockPlatform=arduino
  wires:
  Byte Pack/1 -> Serial Transmit/1
  Data Type Conversion1/1 -> Byte Pack/1
  In1/1 -> Data Type Conversion1/1

== system BalanceCode_MSM_Micro_20b/Plot and Tune Serial0 (USB) or Serial1//Serial2//Serial3 Double Click to Use (2020b and later)/Send//Recieve to Serial0//Serial1//Serial2//Serial3/Serial 2 Send//Recieve/Update  Variables On Status Change ==
  data : Inport
  status : Inport  Port=2
  Delay : Delay  DelayLength=1  InitialCondition=Data0  SampleTime=TS
  MATLAB Function1 : MATLAB Function  TreatAsAtomicUnit=on
  y : Outport
  wires:
  Delay/1 -> MATLAB Function1/2(prev_data)
  MATLAB Function1/1(y) -> Delay/1, y/1
  data/1 -> MATLAB Function1/1(data)
  status/1 -> MATLAB Function1/3(status)

== system BalanceCode_MSM_Micro_20b/Plot and Tune Serial0 (USB) or Serial1//Serial2//Serial3 Double Click to Use (2020b and later)/Send//Recieve to Serial0//Serial1//Serial2//Serial3/Serial 3 Send//Recieve/Send Data To Computer ==
  In1 : Inport
  Enable : EnablePort
  Byte Pack : svdutilitieslib/Byte Pack  maskPackedDataType=uint8  datatypes={'single'}  byteAlign=1  blockPlatform=arduinoert
      settings: SourceProductBaseCode=ANDROID,ARDUINO,ML_ARDUINO,ECCORTEXA,ECCORTEXR,SC_BEAGLEBONE_BLUE,EC_FREEDOM_BOARD,EC_FRDM_K64F,INTEL_BLOCKSET,JETSONCPU,MICROBIT,NUCLEO,NVIDIA,PX4AUTOPILOTS,RASPPIIO,STMICRODIS,TIC2000,XILINX_BLOCKSET
  Data Type Conversion1 : DataTypeConversion  OutDataTypeStr=single
  Serial Transmit : arduinolib/Serial Transmit  portNumber=3  sendmode=write  sendformat=Decimal  floatprecision=2  blockPlatform=arduino
  wires:
  In1/1 -> Data Type Conversion1/1
  Data Type Conversion1/1 -> Byte Pack/1
  Byte Pack/1 -> Serial Transmit/1

== system BalanceCode_MSM_Micro_20b/Plot and Tune Serial0 (USB) or Serial1//Serial2//Serial3 Double Click to Use (2020b and later)/Send//Recieve to Serial0//Serial1//Serial2//Serial3/Serial 3 Send//Recieve/Update  Variables On Status Change ==
  data : Inport
  status : Inport  Port=2
  Delay : Delay  DelayLength=1  InitialCondition=[Data0]  SampleTime=TS
  MATLAB Function1 : MATLAB Function  TreatAsAtomicUnit=on
  y : Outport
  wires:
  status/1 -> MATLAB Function1/3(status)
  data/1 -> MATLAB Function1/1(data)
  MATLAB Function1/1(y) -> y/1, Delay/1
  Delay/1 -> MATLAB Function1/2(prev_data)

== system BalanceCode_MSM_Micro_20b/Subsystem1/Caclulate GyroBias/Caclulate GyroBias/Gyro Calibration Discrete LPF1 ==
  Gyro : Inport
  Discrete-Time Integrator : DiscreteIntegrator  SampleTime=-1  ICPrevOutput=DiscIntNeverNeededParam  ICPrevScaledInput=DiscIntNeverNeededParam
  Gain : Gain  Gain=1/.1
  Sum : Sum  Inputs=|+-
  Out1 : Outport
  wires:
  Sum/1 -> Gain/1
  Gain/1 -> Discrete-Time Integrator/1
  Gyro/1 -> Sum/1
  Discrete-Time Integrator/1 -> Sum/2, Out1/1

== matlab function BalanceCode_MSM_Micro_20b/Plot and Tune Serial0 (USB) or Serial1//Serial2//Serial3 Double Click to Use (2020b and later)/Send//Recieve to Serial0//Serial1//Serial2//Serial3/Serial 1 Send//Recieve/Update  Variables On Status Change/MATLAB Function1 ==
  data: data input; y output; prev_data input; status input
function y= fcn(data,prev_data,status)

if(status)
    y=data;
else
    y=prev_data;
end

== matlab function BalanceCode_MSM_Micro_20b/Plot and Tune Serial0 (USB) or Serial1//Serial2//Serial3 Double Click to Use (2020b and later)/Send//Recieve to Serial0//Serial1//Serial2//Serial3/Serial 2 Send//Recieve/Update  Variables On Status Change/MATLAB Function1 ==
  data: data input; y output; prev_data input; status input
function y= fcn(data,prev_data,status)

if(status)
    y=data;
else
    y=prev_data;
end

== matlab function BalanceCode_MSM_Micro_20b/Plot and Tune Serial0 (USB) or Serial1//Serial2//Serial3 Double Click to Use (2020b and later)/Send//Recieve to Serial0//Serial1//Serial2//Serial3/Serial 3 Send//Recieve/Update  Variables On Status Change/MATLAB Function1 ==
  data: data input; y output; prev_data input; status input
function y= fcn(data,prev_data,status)

if(status)
    y=data;
else
    y=prev_data;
end

== matlab function BalanceCode_MSM_Micro_20b/Plot and Tune Serial0 (USB) or Serial1//Serial2//Serial3 Double Click to Use (2020b and later)/Send//Recieve to Serial0//Serial1//Serial2//Serial3/Serial 0 Send//Recieve/Update  Variables On Status Change/MATLAB Function1 ==
  data: data input; y output; prev_data input; status input
function y= fcn(data,prev_data,status)

if(status)
    y=data;
else
    y=prev_data;
end
